simulink model "HW1_Q3_part4_99101751_99102156"  (R2021a)
settings: Solver=VariableStepAuto  StartTime=0.0  StopTime=10.0  RelTol=1e-3
libraries: dspsrcs4 x1
settings Model: Creator=Gold System 88518747  LastModifiedBy=Gold System 88518747

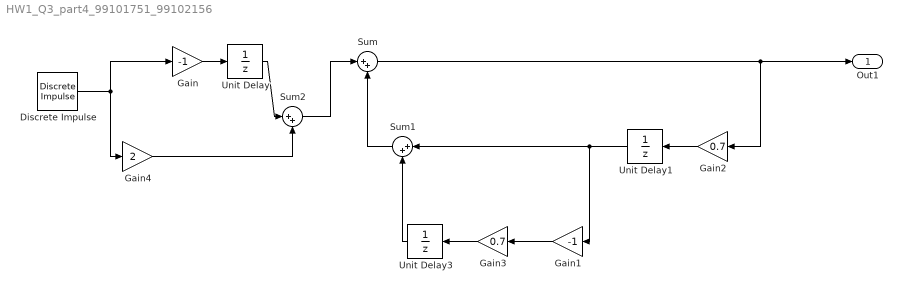
== system HW1_Q3_part4_99101751_99102156 ==
  Discrete Impulse : dspsrcs4/Discrete  Impulse  Delay=0  SampleTime=1  FrameSample=1  OutputFrames=off  dataType=double  isSigned=on  wordLen=16  udDataType=sfix(16)  fracBitsMode=Best precision  numFracBits=15  OutDataTypeStr=double  LastOutDataTypeStr=double
  Gain : Gain  Gain=-1
  Gain1 : Gain  Gain=-1
  Gain2 : Gain  Gain=0.7
  Gain3 : Gain  Gain=0.7
  Gain4 : Gain  Gain=2
  Sum : Sum  Inputs=|++
  Sum1 : Sum  Inputs=|++
  Sum2 : Sum  Inputs=|++
  Unit Delay : UnitDelay  SampleTime=-1  HasFrameUpgradeWarning=on
  Unit Delay1 : UnitDelay  SampleTime=-1  HasFrameUpgradeWarning=on
  Unit Delay3 : UnitDelay  SampleTime=-1  HasFrameUpgradeWarning=on
  Out1 : Outport
  wires:
  Gain/1 -> Unit Delay/1
  Discrete Impulse/1 -> Gain4/1, Gain/1
  Gain2/1 -> Unit Delay1/1
  Sum/1 -> Gain2/1, Out1/1
  Unit Delay1/1 -> Gain1/1, Sum1/1
  Gain3/1 -> Unit Delay3/1
  Gain1/1 -> Gain3/1
  Unit Delay3/1 -> Sum1/2
  Sum1/1 -> Sum/2
  Gain4/1 -> Sum2/2
  Unit Delay/1 -> Sum2/1
  Sum2/1 -> Sum/1
